simulink model "ATRIAS_vnmc"  (R2015a)
settings: Solver=ode45  StartTime=0.0  StopTime=60  FixedStep=1e-3  MinStep=1e-6  RelTol=1e-3  AbsTol=1e-4
values from neighbouring files (symbols this model uses):
  initial_boom_yaw = initial_boom_yaw + delta_yaw0    [run_model.m]
  max_floor_diff = cost_fun_opts.max_floor_diff    [opt_cmaes.m]    (also in run_model.m; set_all_params_simple.m = 0)
  noise_on_off = cost_fun_opts.noise_on_off    [opt_cmaes.m]    (also in run_model.m; set_all_params_simple.m = 0)
  noise_seed = cost_fun_opts.noise_seed    [opt_cmaes.m]    (also in run_model.m; set_all_params_simple.m = 1)
  noise_variance = cost_fun_opts.noise_variance    [opt_cmaes.m]    (also in run_model.m; set_all_params_simple.m = 0.000174532925199)
  SEA_swing_ctrl_on_off = cost_fun_opts.SEA_swing_ctrl_on_off    [opt_cmaes.m]    (also in run_model.m; set_all_params_simple.m = 0)
  sim_t = simout.twalk    [run_model.m]
  steady_dist = cost_fun_opts.steady_dist    [opt_cmaes.m]    (also in run_model.m; set_all_params_simple.m = 10)
  ts_anim = 0.0333    [run_model.m]
undefined symbols (not defined in the file or in its folder): A1_notch_f1, A2_notch_f1, A_lpf_dtau, A_lpf_velocity, B1_lpf_dtau, B1_lpf_velocity, B1_notch_f1, B2_lpf_dtau, B2_lpf_velocity, B2_notch_f1, b_hmotor, b_leg_spring, b_rotor, base_color_d, boom_color_d, boom_mount_to_center_diagonal, breakaway_friction, c, c_jointstop, com_height_offset, contactThr, coulomb_friction, CtrlPar_theta0, D12_S, D12_T, d_com, ddx_max, ddy_max, delta_phi_max, delta_phi_max_buffer, delta_phi_max_dropoff, delta_phi_min, des_forward_velocity, DS_width, dtau_des_max, dtheta0_vmc, dx0_vmc, dy_max, eref, fblink_color_d, fcut_acceleration, floor_color_d, floor_tile_width, floor_zero_height, FmaxBFSH, FmaxGLU, FmaxHAM, FmaxHFL, FmaxRF, FmaxVAS, FPCtrlPar, friction_linear_zone, g, gain_nodes_sea_torque, gamma_stance_thr, gamma_swing_thr, hip_height, HIP_MTR_MAX_CONT_TORQUE, HIP_MTR_MAX_TORQUE, hshaft_color_d ... (+236)
libraries: sm_lib x280, nesl_utility x174, simulink x114, simulink_extras x58, fl_lib x16, mblibv1 x2, dspswit3 x2
(part 10 of 23)

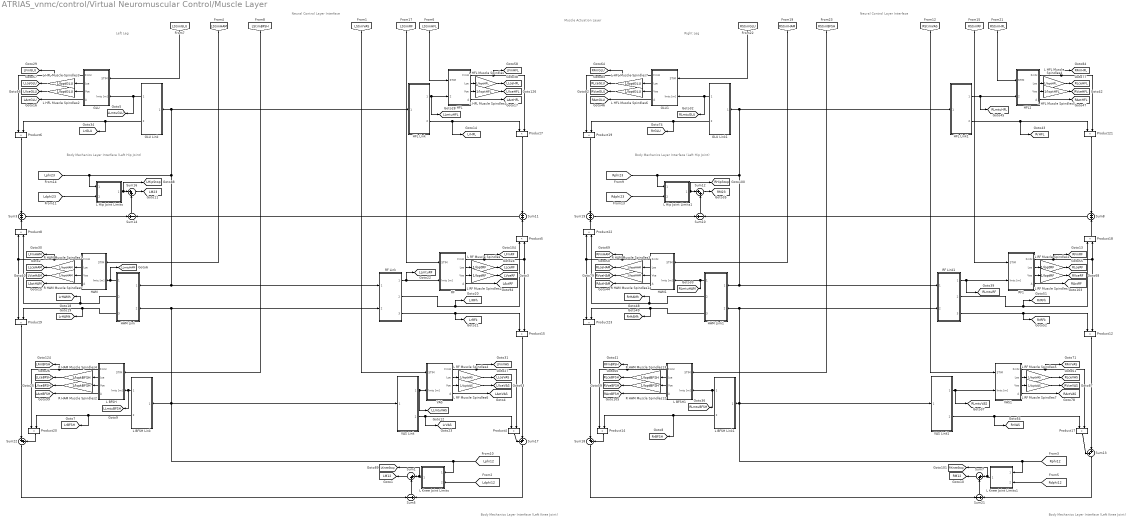
== system ATRIAS_vnmc/control/Virtual Neuromuscular Control/Muscle Layer ==
  note: Left Leg
  note: Neural Control Layer Interface
  note: Muscle Actuation Layer
  note: Body Mechanics Layer
      | Interface (Left Hip Joint)
  note: Body Mechanics Layer
      | Interface (Left Knee Joint)
  note: Right Leg
  note: Neural Control Layer Interface
  note: Body Mechanics Layer
      | Interface (Left Hip Joint)
  note: Body Mechanics Layer
      | Interface (Left Knee Joint)
  GLU : Subsystem
  GLU Link : Subsystem
  GLU Link1 : Subsystem
  GLU1 : Subsystem
  HAM : Subsystem
  HAM Link : Subsystem
  HAM Link1 : Subsystem
  HAM1 : Subsystem
  HFL : Subsystem
  HFL Link : Subsystem
  HFL Link1 : Subsystem
  HFL1 : Subsystem
  L BFSH : Subsystem
  L BFSH Link : Subsystem
  L BFSH Link1 : Subsystem
  L BFSH1 : Subsystem
  L HFL Muscle Spindles{,1,4..5} (4 alike) : Gain  Gain=1/loptHFL
  L HFL Muscle Spindles{2..3,6..7} (4 alike) : Gain  Gain=1/loptGLU
  L Hip Joint Limits : Subsystem
  L Hip Joint Limits1 : Subsystem
  L Knee Joint Limits : Subsystem
  L Knee Joint Limits1 : Subsystem
  L RF Muscle Spindles{,1..3} (4 alike) : Gain  Gain=1/loptRF
  L RF Muscle Spindles{4..7} (4 alike) : Gain  Gain=1/loptVAS
  Product{4..9,12,14..15,17..23} (16 alike) : Product  RndMeth=Zero
  R HAM Muscle Spindles{1,3,6,14} (4 alike) : Gain  Gain=1/loptHAM
  R HAM Muscle Spindles{2,4,12..13} (4 alike) : Gain  Gain=1/loptBFSH
  RF : Subsystem
  RF Link : Subsystem
  RF Link1 : Subsystem
  RF1 : Subsystem
  Sum{1,7,12,16,18,22} (6 alike) : Sum  Inputs=|++
  Sum10 : Sum  Inputs=+-
  Sum{3,8,11,19} (4 alike) : Sum
  Sum13 : Sum  Inputs=++|
  Sum14 : Sum  Inputs=+-
  Sum17 : Sum  Inputs=++|
  Sum21 : Sum  Inputs=-+
  Sum5 : Sum  Inputs=-+
  VAS : Subsystem
  VAS Link : Subsystem
  VAS Link1 : Subsystem
  VAS1 : Subsystem
  tag scope: LActBFSH=global, LActGLU=global, LActHAM=global, LActHFL=global, LActRF=global, LActVAS=global, LFmBFSH=global, LFmGLU=global, LFmHAM=global, LFmHFL=global, LFmRF=global, LFmVAS=global, LHipStop=global, LKneeStop=global, LLceBFSH=global, LLceGLU=global, LLceHAM=global, LLceHFL=global, LLceRF=global, LLceVAS=global, LLmtuBFSH=global, LLmtuGLU=global, LLmtuHAM=global, LLmtuHFL=global, LLmtuRF=global, LLmtuVAS=global, LM12=global, LM23=global, LVceBFSH=global, LVceGLU=global, LVceHAM=global, LVceHFL=global, LVceRF=global, LVceVAS=global, LrBFSH=global, LrGLU=global, LrHAMh=global, LrHAMk=global, LrHFL=global, LrRFh=global, LrRFk=global, LrVAS=global, RActBFSH=global, RActGLU=global, RActHAM=global, RActHFL=global, RActRF=global, RActVAS=global, RFmBFSH=global, RFmGLU=global, RFmHAM=global, RFmHFL=global, RFmRF=global, RFmVAS=global, RHipStop=global, RKneeStop=global, RLceBFSH=global, RLceGLU=global, RLceHAM=global, RLceHFL=global, RLceRF=global, RLceVAS=global, RLmtuBFSH=global, RLmtuGLU=global, RLmtuHAM=global, RLmtuHFL=global, RLmtuRF=global, RLmtuVAS=global, RM12=global, RM23=global, RVceBFSH=global, RVceGLU=global, RVceHAM=global, RVceHFL=global, RVceRF=global, RVceVAS=global, RrBFSH=global, RrGLU=global, RrHAMh=global, RrHAMk=global, RrHFL=global, RrRFh=global, RrRFk=global, RrVAS=global
  wires:
  [Lphi12] -> L Knee Joint Limits/1(phi [rad]1), VAS Link/1(phi23 [rad]), RF Link/2(phi23 [rad]), HAM Link/2(phi23 [rad]), L BFSH Link/1(phi23 [rad])
  [LStimHAM] -> HAM/1(STIM)
  HAM/1(Fmtc) -> Product9/1, Product8/1, [LFmHAM]
  HAM/2(Lce) -> R HAM Muscle Spindles1/1
  HFL/1(Fmtc) -> Product7/2, [LFmHFL]
  HFL/2(Lce) -> L HFL Muscle Spindles/1
  [LStimHFL] -> HFL/1(STIM)
  GLU/1(Fmtc) -> Product6/1, [LFmGLU]
  [LStimGLU] -> GLU/1(STIM)
  Sum16/1 -> [LM23]
  [Ldphi12] -> L Knee Joint Limits/2(dphi [rad/s]1)
  VAS Link/1(lmtu [m]) -> [LLmtuVAS], VAS/2(lmtc [m])
  HAM Link/1(lmtu [m]) -> [LLmtuHAM], HAM/2(lmtc [m])
  HAM Link/2(lever34 [m]) -> Product8/2, [LrHAMh]
  HAM Link/3(lever23 [m]) -> Product9/2, [LrHAMk]
  Sum3/1 -> Sum14/1
  [Lphi23] -> L Hip Joint Limits/1(phi [rad]1), HFL Link/1(phi34 [rad]), GLU Link/1(phi34 [rad]), RF Link/1(phi34 [rad]), HAM Link/1(phi34 [rad])
  VAS/4(A) -> [LActVAS]
  VAS/1(Fmtc) -> Product4/2, [LFmVAS]
  Sum1/1 -> [LM12]
  L Knee Joint Limits/1(M_stop [Nm]1) -> Sum1/1, [LKneeStop]
  Sum5/1 -> Sum1/2
  VAS Link/2(lever [m]) -> [LrVAS], Product4/1
  Sum22/1 -> Sum5/1
  HAM/4(A) -> [LActHAM]
  Product8/1 -> Sum3/2
  Product6/1 -> Sum3/1
  GLU Link/1(lmtu [m]) -> [LLmtuGLU], GLU/2(lmtc [m])
  GLU Link/2(lever [m]) -> Product6/2, [LrGLU]
  GLU/4(A) -> [LActGLU]
  [Ldphi23] -> L Hip Joint Limits/2(dphi [rad/s]1)
  L Hip Joint Limits/1(M_stop [Nm]1) -> [LHipStop], Sum16/1
  Sum14/1 -> Sum16/2
  HFL Link/1(lmtu [m]) -> [LLmtuHFL], HFL/2(lmtc [m])
  HFL/4(A) -> [LActHFL]
  HFL Link/2(lever [m]) -> Product7/1, [LrHFL]
  [LStimVAS] -> VAS/1(STIM)
  GLU/2(Lce) -> L HFL Muscle Spindles3/1
  GLU/3(Vce) -> L HFL Muscle Spindles2/1
  HAM/3(Vce) -> R HAM Muscle Spindles6/1
  VAS/3(Vce) -> L RF Muscle Spindles6/1
  VAS/2(Lce) -> L RF Muscle Spindles4/1
  HFL/3(Vce) -> L HFL Muscle Spindles1/1
  RF/4(A) -> [LActRF]
  RF/3(Vce) -> L RF Muscle Spindles2/1
  RF/2(Lce) -> L RF Muscle Spindles/1
  RF Link/1(lmtu [m]) -> [LLmtuRF], RF/2(lmtc [m])
  RF Link/2(lever34 [m]) -> Product5/1, [LrRFh]
  RF Link/3(lever23 [m]) -> Product15/1, [LrRFk]
  [LStimRF] -> RF/1(STIM)
  Product7/1 -> Sum11/1
  Product5/1 -> Sum11/2
  Product15/1 -> Sum17/2
  Sum17/1 -> Sum5/2
  Product4/1 -> Sum17/1
  [LStimBFSH] -> L BFSH/1(STIM)
  L BFSH Link/1(lmtu [m]) -> [LLmtuBFSH], L BFSH/2(lmtc [m])
  L BFSH Link/2(lever [m]) -> [LrBFSH], Product20/2
  L BFSH/4(A) -> [LActBFSH]
  L BFSH/2(Lce) -> R HAM Muscle Spindles4/1
  L BFSH/3(Vce) -> R HAM Muscle Spindles2/1
  Product20/1 -> Sum22/2
  Product9/1 -> Sum22/1
  L HFL Muscle Spindles1/1 -> [LVceHFL]
  L HFL Muscle Spindles2/1 -> [LVceGLU]
  L HFL Muscle Spindles3/1 -> [LLceGLU]
  L RF Muscle Spindles6/1 -> [LVceVAS]
  RF/1(Fmtc) -> Product5/2, Product15/2, [LFmRF]
  L BFSH/1(Fmtc) -> Product20/1, [LFmBFSH]
  L HFL Muscle Spindles/1 -> [LLceHFL]
  R HAM Muscle Spindles1/1 -> [LLceHAM]
  R HAM Muscle Spindles6/1 -> [LVceHAM]
  L RF Muscle Spindles/1 -> [LLceRF]
  L RF Muscle Spindles2/1 -> [LVceRF]
  R HAM Muscle Spindles4/1 -> [LLceBFSH]
  R HAM Muscle Spindles2/1 -> [LVceBFSH]
  L RF Muscle Spindles4/1 -> [LLceVAS]
  [Rphi12] -> L Knee Joint Limits1/1(phi [rad]1), VAS Link1/1(phi23 [rad]), HAM Link1/2(phi23 [rad]), RF Link1/2(phi23 [rad]), L BFSH Link1/1(phi23 [rad])
  [RStimHAM] -> HAM1/1(STIM)
  HAM1/1(Fmtc) -> Product23/1, Product22/1, [RFmHAM]
  HAM1/2(Lce) -> R HAM Muscle Spindles3/1
  HFL1/1(Fmtc) -> Product21/2, [RFmHFL]
  HFL1/2(Lce) -> L HFL Muscle Spindles4/1
  [RStimHFL] -> HFL1/1(STIM)
  GLU1/1(Fmtc) -> Product19/1, [RFmGLU]
  [RStimGLU] -> GLU1/1(STIM)
  Sum12/1 -> [RM23]
  [Rdphi12] -> L Knee Joint Limits1/2(dphi [rad/s]1)
  VAS Link1/1(lmtu [m]) -> [RLmtuVAS], VAS1/2(lmtc [m])
  HAM Link1/1(lmtu [m]) -> [RLmtuHAM], HAM1/2(lmtc [m])
  HAM Link1/2(lever34 [m]) -> Product22/2, [RrHAMh]
  HAM Link1/3(lever23 [m]) -> Product23/2, [RrHAMk]
  Sum19/1 -> Sum10/1
  [Rphi23] -> L Hip Joint Limits1/1(phi [rad]1), HFL Link1/1(phi34 [rad]), GLU Link1/1(phi34 [rad]), RF Link1/1(phi34 [rad]), HAM Link1/1(phi34 [rad])
  VAS1/4(A) -> [RActVAS]
  VAS1/1(Fmtc) -> Product17/2, [RFmVAS]
  Sum7/1 -> [RM12]
  L Knee Joint Limits1/1(M_stop [Nm]1) -> Sum7/1, [RKneeStop]
  Sum21/1 -> Sum7/2
  VAS Link1/2(lever [m]) -> [RrVAS], Product17/1
  Sum18/1 -> Sum21/1
  HAM1/4(A) -> [RActHAM]
  Product22/1 -> Sum19/2
  Product19/1 -> Sum19/1
  GLU Link1/1(lmtu [m]) -> [RLmtuGLU], GLU1/2(lmtc [m])
  GLU Link1/2(lever [m]) -> Product19/2, [RrGLU]
  GLU1/4(A) -> [RActGLU]
  [Rdphi23] -> L Hip Joint Limits1/2(dphi [rad/s]1)
  L Hip Joint Limits1/1(M_stop [Nm]1) -> [RHipStop], Sum12/1
  Sum10/1 -> Sum12/2
  HFL Link1/1(lmtu [m]) -> [RLmtuHFL], HFL1/2(lmtc [m])
  HFL1/4(A) -> [RActHFL]
  HFL Link1/2(lever [m]) -> Product21/1, [RrHFL]
  [RStimVAS] -> VAS1/1(STIM)
  GLU1/2(Lce) -> L HFL Muscle Spindles7/1
  GLU1/3(Vce) -> L HFL Muscle Spindles6/1
  HAM1/3(Vce) -> R HAM Muscle Spindles14/1
  VAS1/3(Vce) -> L RF Muscle Spindles7/1
  VAS1/2(Lce) -> L RF Muscle Spindles5/1
  HFL1/3(Vce) -> L HFL Muscle Spindles5/1
  RF1/4(A) -> [RActRF]
  RF1/3(Vce) -> L RF Muscle Spindles3/1
  RF1/2(Lce) -> L RF Muscle Spindles1/1
  RF Link1/1(lmtu [m]) -> [RLmtuRF], RF1/2(lmtc [m])
  RF Link1/2(lever34 [m]) -> Product18/1, [RrRFh]
  RF Link1/3(lever23 [m]) -> [RrRFk], Product12/1
  [RStimRF] -> RF1/1(STIM)
  Sum8/1 -> Sum10/2
  Product21/1 -> Sum8/1
  Product18/1 -> Sum8/2
  Product12/1 -> Sum13/2
  Sum13/1 -> Sum21/2
  Product17/1 -> Sum13/1
  [RStimBFSH] -> L BFSH1/1(STIM)
  L BFSH Link1/1(lmtu [m]) -> [RLmtuBFSH], L BFSH1/2(lmtc [m])
  L BFSH Link1/2(lever [m]) -> [RrBFSH], Product14/2
  L BFSH1/4(A) -> [RActBFSH]
  L BFSH1/2(Lce) -> R HAM Muscle Spindles13/1
  L BFSH1/3(Vce) -> R HAM Muscle Spindles12/1
  Product14/1 -> Sum18/2
  Product23/1 -> Sum18/1
  L HFL Muscle Spindles5/1 -> [RVceHFL]
  L HFL Muscle Spindles6/1 -> [RVceGLU]
  L HFL Muscle Spindles7/1 -> [RLceGLU]
  L RF Muscle Spindles7/1 -> [RVceVAS]
  RF1/1(Fmtc) -> Product18/2, Product12/2, [RFmRF]
  L BFSH1/1(Fmtc) -> Product14/1, [RFmBFSH]
  L HFL Muscle Spindles4/1 -> [RLceHFL]
  R HAM Muscle Spindles3/1 -> [RLceHAM]
  R HAM Muscle Spindles14/1 -> [RVceHAM]
  L RF Muscle Spindles1/1 -> [RLceRF]
  L RF Muscle Spindles3/1 -> [RVceRF]
  R HAM Muscle Spindles13/1 -> [RLceBFSH]
  R HAM Muscle Spindles12/1 -> [RVceBFSH]
  L RF Muscle Spindles5/1 -> [RLceVAS]
  Sum11/1 -> Sum14/2

== system ATRIAS_vnmc/control/Virtual Neuromuscular Control/Neural Control Layer1 ==
  note: Neural Control Layer
      | (Sagittal Plane)
  Add{1..3,9} (4 alike) : Sum  Inputs=2
  Add4 : Sum  Inputs=4
  Add5 : Sum  Inputs=4
  Data Type Conversion : DataTypeConversion  OutDataTypeStr=boolean
  Data Type Conversion1 : DataTypeConversion  OutDataTypeStr=boolean
  Demux3 : Demux  Outputs=6
  Demux4 : Demux  Outputs=6
  L Stance Phase (sagittal) : Subsystem  TreatAsAtomicUnit=on
  "L Stance, Swing, Trans (sagittal)" : Subsystem
  L Swing Phase (sagittal) : Subsystem  TreatAsAtomicUnit=on
  Logical Operator : Logic  Operator=NOT  AllPortsSameDT=off  OutDataTypeStr=boolean
  Logical Operator1 : Logic  Operator=NOT  AllPortsSameDT=off  OutDataTypeStr=boolean
  Logical Operator2 : Logic  Operator=OR  AllPortsSameDT=off  OutDataTypeStr=boolean
  Logical Operator3 : Logic  Operator=OR  AllPortsSameDT=off  OutDataTypeStr=boolean
  MDelay{1..4} (4 alike) : Delay  DelayLength=MidDelay_discrete  InitialCondition=0  SampleTime=sample_time
  Mux : Mux  Inputs=6
  Mux1 : Mux  Inputs=6
  Mux2 : Mux  Inputs=2
  Mux4 : Mux  Inputs=2
  R Stance Phase (sagittal) : Subsystem  TreatAsAtomicUnit=on
  "R Stance, Swing, Trans (sagittal)" : Subsystem
  R Swing Phase (sagittal) : Subsystem  TreatAsAtomicUnit=on
  Saturation1 : Saturate  UpperLimit=1  LowerLimit=0.01  ZeroCross=off
  Saturation10 : Saturate  UpperLimit=1  LowerLimit=0.01  ZeroCross=off
  Sum1 : Sum  Inputs=-+|
  Sum6 : Sum  Inputs=-+|
  hipM{1,4,8..9,11..12} (6 alike) : Selector  InputPortWidth=2
  hipM10 : Selector  InputPortWidth=3  Indices=2
  hipM13 : Selector  InputPortWidth=3  Indices=3
  hipM{3,6,14..15,17..18} (6 alike) : Selector  InputPortWidth=2  Indices=2
  hipM16 : Selector  InputPortWidth=3  Indices=3
  hipM2 : Selector  InputPortWidth=3
  hipM5 : Selector  InputPortWidth=3
  hipM7 : Selector  InputPortWidth=3  Indices=2
  tag scope: LAct=global, LHSwStim=global, LStance=global, LStimBFSH=global, LStimGLU=global, LStimHAM=global, LStimHFL=global, LStimRF=global, LStimVAS=global, LSwingPhase=global, RAct=global, RHSwStim=global, RStance=global, RStimBFSH=global, RStimGLU=global, RStimHAM=global, RStimHFL=global, RStimRF=global, RStimVAS=global, RSwingPhase=global
  wires:
  MDelay4/1 -> R Stance Phase (sagittal)/5(FmVAS)
  MDelay3/1 -> L Stance Phase (sagittal)/5(FmVAS)
  [RStance] -> "L Stance, Swing, Trans (sagittal)"/3(CStance)
  [RFootCnt] -> Data Type Conversion1/1
  [LFootCnt] -> Data Type Conversion/1
  [Rphi12] -> R Swing Phase (sagittal)/7(phiK)
  [Rphi23] -> R Swing Phase (sagittal)/6(phiH)
  [Rdphi12] -> R Swing Phase (sagittal)/8(dphiK)
  [Rdalpha] -> R Swing Phase (sagittal)/5(da)
  [Ralpha] -> R Swing Phase (sagittal)/4(a)
  [RLength] -> R Swing Phase (sagittal)/10(l)
  Sum1/1 -> R Swing Phase (sagittal)/3(a_tgt)
  [theta] -> Sum1/1
  [Ralpha_tgt] -> Sum1/2
  [leg_clr] -> R Swing Phase (sagittal)/9(l_clr)
  [Lphi12] -> L Swing Phase (sagittal)/7(phiK)
  [Lphi23] -> L Swing Phase (sagittal)/6(phiH)
  [Ldphi12] -> L Swing Phase (sagittal)/8(dphiK)
  [Ldalpha] -> L Swing Phase (sagittal)/5(da)
  [Lalpha] -> L Swing Phase (sagittal)/4(a)
  [LLength] -> L Swing Phase (sagittal)/10(l)
  Add5/1 -> Mux1/6  "BFSH"
  hipM18/1 -> Add5/4
  hipM17/1 -> Add5/3
  R Swing Phase (sagittal)/3(S_M7_DS [BFSH]) -> Add5/1, "R Stance, Swing, Trans (sagittal)"/14(S_M7_DS)
  hipM16/1 -> Mux1/5  "VAS"
  R Swing Phase (sagittal)/7(M10 [HFL GLU VAS]) -> hipM10/1, hipM2/1, "R Stance, Swing, Trans (sagittal)"/18(S_M10), hipM16/1
  R Swing Phase (sagittal)/5(M8 [RF BFSH]) -> hipM17/1, hipM12/1, "R Stance, Swing, Trans (sagittal)"/16(S_M8)
  R Swing Phase (sagittal)/4(S_M7_Sw [BFSH]) -> Add5/2, "R Stance, Swing, Trans (sagittal)"/15(S_M7_Sw)
  hipM15/1 -> Add4/4
  hipM14/1 -> Add4/3
  L Swing Phase (sagittal)/3(S_M7_DS [BFSH]) -> "L Stance, Swing, Trans (sagittal)"/14(S_M7_DS), Add4/1
  Add4/1 -> Mux/6  "BFSH"
  hipM13/1 -> Mux/5  "VAS"
  "L Stance, Swing, Trans (sagittal)"/2(S_Modules) -> [LAct]
  "R Stance, Swing, Trans (sagittal)"/2(S_Modules) -> [RAct]
  R Swing Phase (sagittal)/8(Phase [M7 M8 M9 M10]) -> [RSwingPhase]
  L Swing Phase (sagittal)/8(Phase [M7 M8 M9 M10]) -> [LSwingPhase]
  hipM11/1 -> Mux1/4  "HAM"
  hipM12/1 -> Mux1/3  "RF"
  Add2/1 -> Mux1/2  "GLU"
  hipM10/1 -> Add2/2
  hipM3/1 -> Add2/1
  Add3/1 -> Mux1/1  "HFL"
  hipM2/1 -> Add3/2
  hipM1/1 -> Add3/1
  Mux1/1 -> [RHSwStim]
  R Swing Phase (sagittal)/6(M9 [HAM BFSH]) -> hipM18/1, hipM11/1, "R Stance, Swing, Trans (sagittal)"/17(S_M9)
  R Swing Phase (sagittal)/2(S_M6 [HFL GLU]) -> hipM1/1, hipM3/1, "R Stance, Swing, Trans (sagittal)"/13(S_M6)
  R Swing Phase (sagittal)/1(S_Sw_0) -> "R Stance, Swing, Trans (sagittal)"/12(S_0_Sw)
  "R Stance, Swing, Trans (sagittal)"/1(S) -> Saturation1/1
  hipM8/1 -> Mux/4  "HAM"
  hipM9/1 -> Mux/3  "RF"
  Add1/1 -> Mux/2  "GLU"
  hipM7/1 -> Add1/2
  hipM6/1 -> Add1/1
  Add9/1 -> Mux/1  "HFL"
  hipM5/1 -> Add9/2
  hipM4/1 -> Add9/1
  Mux/1 -> [LHSwStim]
  L Swing Phase (sagittal)/7(M10 [HFL GLU VAS]) -> hipM7/1, hipM5/1, "L Stance, Swing, Trans (sagittal)"/18(S_M10), hipM13/1
  L Swing Phase (sagittal)/6(M9 [HAM BFSH]) -> hipM8/1, "L Stance, Swing, Trans (sagittal)"/17(S_M9), hipM15/1
  L Swing Phase (sagittal)/5(M8 [RF BFSH]) -> hipM14/1, hipM9/1, "L Stance, Swing, Trans (sagittal)"/16(S_M8)
  L Swing Phase (sagittal)/4(S_M7_Sw [BFSH]) -> "L Stance, Swing, Trans (sagittal)"/15(S_M7_Sw), Add4/2
  L Swing Phase (sagittal)/2(S_M6 [HFL GLU]) -> "L Stance, Swing, Trans (sagittal)"/13(S_M6), hipM4/1, hipM6/1
  L Stance Phase (sagittal)/5(S_M4 [HFL GLU HAM]) -> "L Stance, Swing, Trans (sagittal)"/11(S_M4)
  R Stance Phase (sagittal)/5(S_M4 [HFL GLU HAM]) -> "R Stance, Swing, Trans (sagittal)"/11(S_M4)
  Mux4/1 -> R Stance Phase (sagittal)/3(theta dtheta [rad rad/s])
  Mux2/1 -> L Stance Phase (sagittal)/3(theta dtheta [rad rad/s])
  [RLLoad] -> "R Stance, Swing, Trans (sagittal)"/5(ILLoad)
  R Stance Phase (sagittal)/4(S_M3 [HFL GLU HAM]) -> "R Stance, Swing, Trans (sagittal)"/10(S_M3)
  L Stance Phase (sagittal)/4(S_M3 [HFL GLU HAM]) -> "L Stance, Swing, Trans (sagittal)"/10(S_M3)
  [theta_tgt] -> R Stance Phase (sagittal)/2(theta_tgt [rad])
  [dtheta] -> Mux4/2
  [theta] -> Mux4/1
  [LLLoad] -> "L Stance, Swing, Trans (sagittal)"/5(ILLoad)
  [theta_tgt] -> L Stance Phase (sagittal)/2(theta_tgt [rad])
  [dtheta] -> Mux2/2
  [theta] -> Mux2/1
  R Stance Phase (sagittal)/3(S_M2 [VAS BFSH]) -> "R Stance, Swing, Trans (sagittal)"/9(S_M2)
  R Stance Phase (sagittal)/2(S_M1 [VAS]) -> "R Stance, Swing, Trans (sagittal)"/8(S_M1)
  L Stance Phase (sagittal)/3(S_M2 [VAS BFSH]) -> "L Stance, Swing, Trans (sagittal)"/9(S_M2)
  L Stance Phase (sagittal)/2(S_M1 [VAS]) -> "L Stance, Swing, Trans (sagittal)"/8(S_M1)
  R Stance Phase (sagittal)/1(S_St_0) -> "R Stance, Swing, Trans (sagittal)"/7(S_0_St)
  L Swing Phase (sagittal)/1(S_Sw_0) -> "L Stance, Swing, Trans (sagittal)"/12(S_0_Sw)
  L Stance Phase (sagittal)/1(S_St_0) -> "L Stance, Swing, Trans (sagittal)"/7(S_0_St)
  Sum6/1 -> L Swing Phase (sagittal)/3(a_tgt)
  [LStance] -> "R Stance, Swing, Trans (sagittal)"/3(CStance)
  [RStance] -> "R Stance, Swing, Trans (sagittal)"/2(Stance)
  [LStance] -> "L Stance, Swing, Trans (sagittal)"/2(Stance)
  [theta] -> Sum6/1
  [Lalpha_tgt] -> Sum6/2
  Demux4/6 -> [RStimBFSH]
  Demux4/5 -> [RStimVAS]
  Demux4/4 -> [RStimRF]
  Demux4/3 -> [RStimHAM]
  Demux4/2 -> [RStimGLU]
  Demux4/1 -> [RStimHFL]
  Demux3/6 -> [LStimBFSH]
  Demux3/5 -> [LStimVAS]
  Demux3/4 -> [LStimRF]
  Demux3/3 -> [LStimHAM]
  Demux3/2 -> [LStimGLU]
  Demux3/1 -> [LStimHFL]
  [RLLoad] -> "L Stance, Swing, Trans (sagittal)"/6(CLLoad)
  [LonR] -> "R Stance, Swing, Trans (sagittal)"/4(ConI)
  Saturation1/1 -> Demux4/1
  [LLLoad] -> "R Stance, Swing, Trans (sagittal)"/6(CLLoad)
  [TrCtrlPar] -> "R Stance, Swing, Trans (sagittal)"/1(CtrlPar)
  [LonR] -> Logical Operator2/1
  Logical Operator2/1 -> R Swing Phase (sagittal)/Enable
  Logical Operator1/1 -> Logical Operator2/2
  Data Type Conversion1/1 -> [RStance], R Stance Phase (sagittal)/Enable, Logical Operator1/1, R Swing Phase (sagittal)/2(Stance)
  [SwCtrlPar] -> R Swing Phase (sagittal)/1(CtrlPar)
  [RLceBFSH] -> R Stance Phase (sagittal)/6(LceBFSH)
  MDelay1/1 -> MDelay4/1
  [RFmVAS] -> MDelay1/1
  [LHSwStim] -> R Stance Phase (sagittal)/4(CStim_HSw)
  [StCtrlPar] -> R Stance Phase (sagittal)/1(CtrlPar)
  [RonL] -> "L Stance, Swing, Trans (sagittal)"/4(ConI)
  "L Stance, Swing, Trans (sagittal)"/1(S) -> Saturation10/1
  Saturation10/1 -> Demux3/1
  [TrCtrlPar] -> "L Stance, Swing, Trans (sagittal)"/1(CtrlPar)
  [leg_clr] -> L Swing Phase (sagittal)/9(l_clr)
  [RonL] -> Logical Operator3/1
  Logical Operator3/1 -> L Swing Phase (sagittal)/Enable
  Logical Operator/1 -> Logical Operator3/2
  Data Type Conversion/1 -> [LStance], L Stance Phase (sagittal)/Enable, Logical Operator/1, L Swing Phase (sagittal)/2(Stance)
  [SwCtrlPar] -> L Swing Phase (sagittal)/1(CtrlPar)
  [LLceBFSH] -> L Stance Phase (sagittal)/6(LceBFSH)
  MDelay2/1 -> MDelay3/1
  [LFmVAS] -> MDelay2/1
  [RHSwStim] -> L Stance Phase (sagittal)/4(CStim_HSw)
  [StCtrlPar] -> L Stance Phase (sagittal)/1(CtrlPar)

== system ATRIAS_vnmc/control/Virtual Neuromuscular Control/Torque Distribution ==
  note: J^(-T) [tauB; tauF] = [tauH, tauK]
  note: Map Torques
  note: J^(-T) [tauB; tauF] = [tauH, tauK]
  R tauK_des [Nm] : Inport
  R tauH_des [Nm] : Inport  Port=2
  R Jacobian Constant (k) : Inport  Port=3
  L tauK_des [Nm] : Inport  Port=4
  L tauH_des [Nm] : Inport  Port=5
  L Jacobian Constant (k) : Inport  Port=6
  Demux : Demux
  Demux1 : Demux  Outputs=2
  Demux2 : Demux  Outputs=2
  Mux : Mux
  Mux1 : Mux  Inputs=2
  Mux2 : Mux  Inputs=2
  Switch1 : Switch  Criteria=u2 > Threshold
  Switch2 : Switch  Criteria=u2 > Threshold
  Torque Limiter (outside) 1 : Saturate  UpperLimit=max_sagittal_loaded_torque  LowerLimit=-max_sagittal_loaded_torque
      settings: AttributesFormatString=Hi: %<UpperLimit>\nLo: %<LowerLimit>
  Torque Limiter (outside) 2 : Saturate  UpperLimit=max_sagittal_loaded_torque  LowerLimit=-max_sagittal_loaded_torque
      settings: AttributesFormatString=Hi: %<UpperLimit>\nLo: %<LowerLimit>
  Torque Limiter (outside) 3 : Saturate  UpperLimit=max_sagittal_unloaded_torque  LowerLimit=-max_sagittal_unloaded_torque
      settings: AttributesFormatString=Hi: %<UpperLimit>\nLo: %<LowerLimit>
  Torque Limiter (outside) 4 : Saturate  UpperLimit=max_sagittal_unloaded_torque  LowerLimit=-max_sagittal_unloaded_torque
      settings: AttributesFormatString=Hi: %<UpperLimit>\nLo: %<LowerLimit>
  map_tau_L : MATLAB Function  TreatAsAtomicUnit=on
  map_tau_R : MATLAB Function  TreatAsAtomicUnit=on
  mech limit avoidance1 : Subsystem  Commented=on
  R tauB [Nm] : Outport
  R tauF [Nm] : Outport  Port=2
  R J_inv_transpose [2x2] : Outport  Port=3
  L tauB [Nm] : Outport  Port=4
  L tauF [Nm] : Outport  Port=5
  L J_inv_transpose [2x2] : Outport  Port=6
  wires:
  R Jacobian Constant (k)/1 -> map_tau_R/3(k)
  map_tau_R/3(Jinv_trans) -> R J_inv_transpose [2x2]/1
  L Jacobian Constant (k)/1 -> map_tau_L/3(k)
  map_tau_L/3(Jinv_trans) -> L J_inv_transpose [2x2]/1
  map_tau_L/1(tauB) -> Mux2/1
  map_tau_L/2(tauF) -> Mux2/2
  Mux/1 -> Demux/1
  Demux/1 -> [RtauH]
  R tauH_des [Nm]/1 -> Mux/1
  R tauK_des [Nm]/1 -> Mux/2
  L tauH_des [Nm]/1 -> Mux/3
  L tauK_des [Nm]/1 -> Mux/4
  Demux/2 -> [RtauK]
  Demux/3 -> [LtauH]
  Demux/4 -> [LtauK]
  [RtauH] -> map_tau_R/1(tauH_des)
  [RtauK] -> map_tau_R/2(tauK_des)
  [LtauH] -> map_tau_L/1(tauH_des)
  [LtauK] -> map_tau_L/2(tauK_des)
  Switch1/1 -> Demux1/1
  [LFootCnt] -> Switch1/2
  Mux2/1 -> Torque Limiter (outside) 1/1, Torque Limiter (outside) 3/1
  Torque Limiter (outside) 3/1 -> Switch1/3
  Torque Limiter (outside) 1/1 -> Switch1/1
  Demux1/2 -> L tauF [Nm]/1
  Demux1/1 -> L tauB [Nm]/1
  map_tau_R/1(tauB) -> Mux1/1
  map_tau_R/2(tauF) -> Mux1/2
  Switch2/1 -> Demux2/1
  [RFootCnt] -> Switch2/2
  Mux1/1 -> Torque Limiter (outside) 2/1, Torque Limiter (outside) 4/1
  Torque Limiter (outside) 4/1 -> Switch2/3
  Torque Limiter (outside) 2/1 -> Switch2/1
  Demux2/2 -> R tauF [Nm]/1
  Demux2/1 -> R tauB [Nm]/1

== system ATRIAS_vnmc/atrias_system/ATRIAS Mechanical System Layer/Boom/Frame Data ==
  Mux : Mux  Inputs=3
  PS-Simulink Converter{,1..3} (4 alike) : nesl_utility/PS-Simulink Converter  PhysicalDomain=network_engine_domain  SubClassName=ps_output  LeftPortType=input  RightPortType=output  PseudoPeriodic=off  Frequencies=[]  Unit=1  AffineConversion=off
  Transform Sensor : sm_lib/Frames and Transforms/Transform Sensor  MeasurementFrame=World  SenseAngle=off  SenseAxis=off  SenseAngle1=off  SenseAngle2=off  SenseAngle3=off  SenseQ=on  SenseR=off  SenseOmegaX=off  SenseOmegaY=off  SenseOmegaZ=off  SenseOmega1=off  SenseOmega2=off  SenseOmega3=off  SenseQDot=off  SenseRDot=off  SenseAlphaX=off  SenseAlphaY=off  SenseAlphaZ=off  SenseAlpha1=off  SenseAlpha2=off  SenseAlpha3=off  SenseQDDot=off  SenseRDDot=off  SenseX=on  SenseY=on  SenseZ=on  SenseRad=off  SenseAzim=off  SenseDist=off  SenseInc=off  SenseXDot=off  SenseYDot=off  SenseZDot=off  SenseRadDot=off  SenseAzimDot=off  SenseDistDot=off  SenseIncDot=off  SenseXDDot=off  SenseYDDot=off  SenseZDDot=off  SenseRadDDot=off  SenseAzimDDot=off  SenseDistDDot=off  SenseIncDDot=off  BlockFunction=simmechanics.library.frames_transforms.transform_sensor
  World Frame : sm_lib/Frames and Transforms/World Frame  BlockFunction=simmechanics.library.frames_transforms.world_frame
  Frame : PMIOPort  Port=1  Side=Left
  tag scope: QBoom=global, xyzBoom=global
  wires:
  PS-Simulink Converter/1 -> [QBoom]
  PS-Simulink Converter1/1 -> Mux/1
  PS-Simulink Converter2/1 -> Mux/2
  PS-Simulink Converter3/1 -> Mux/3
  Mux/1 -> [xyzBoom]
  connections:
  Transform Sensor/RConn1 -- Frame/RConn1
  Transform Sensor/LConn1 -- World Frame/RConn1
  Transform Sensor/RConn4 -- PS-Simulink Converter2/LConn1
  Transform Sensor/RConn5 -- PS-Simulink Converter3/LConn1
  Transform Sensor/RConn3 -- PS-Simulink Converter1/LConn1
  Transform Sensor/RConn2 -- PS-Simulink Converter/LConn1

== system ATRIAS_vnmc/atrias_system/ATRIAS Mechanical System Layer/Boom Base/Frame Data ==
  Mux : Mux  Inputs=3
  PS-Simulink Converter{,1..3} (4 alike) : nesl_utility/PS-Simulink Converter  PhysicalDomain=network_engine_domain  SubClassName=ps_output  LeftPortType=input  RightPortType=output  PseudoPeriodic=off  Frequencies=[]  Unit=1  AffineConversion=off
  Transform Sensor : sm_lib/Frames and Transforms/Transform Sensor  MeasurementFrame=World  SenseAngle=off  SenseAxis=off  SenseAngle1=off  SenseAngle2=off  SenseAngle3=off  SenseQ=on  SenseR=off  SenseOmegaX=off  SenseOmegaY=off  SenseOmegaZ=off  SenseOmega1=off  SenseOmega2=off  SenseOmega3=off  SenseQDot=off  SenseRDot=off  SenseAlphaX=off  SenseAlphaY=off  SenseAlphaZ=off  SenseAlpha1=off  SenseAlpha2=off  SenseAlpha3=off  SenseQDDot=off  SenseRDDot=off  SenseX=on  SenseY=on  SenseZ=on  SenseRad=off  SenseAzim=off  SenseDist=off  SenseInc=off  SenseXDot=off  SenseYDot=off  SenseZDot=off  SenseRadDot=off  SenseAzimDot=off  SenseDistDot=off  SenseIncDot=off  SenseXDDot=off  SenseYDDot=off  SenseZDDot=off  SenseRadDDot=off  SenseAzimDDot=off  SenseDistDDot=off  SenseIncDDot=off  BlockFunction=simmechanics.library.frames_transforms.transform_sensor
  World Frame : sm_lib/Frames and Transforms/World Frame  BlockFunction=simmechanics.library.frames_transforms.world_frame
  Frame : PMIOPort  Port=1  Side=Left
  tag scope: QBoomBase=global, xyzBoomBase=global
  wires:
  PS-Simulink Converter/1 -> [QBoomBase]
  PS-Simulink Converter1/1 -> Mux/1
  PS-Simulink Converter2/1 -> Mux/2
  PS-Simulink Converter3/1 -> Mux/3
  Mux/1 -> [xyzBoomBase]
  connections:
  PS-Simulink Converter3/LConn1 -- Transform Sensor/RConn5
  PS-Simulink Converter2/LConn1 -- Transform Sensor/RConn4
  PS-Simulink Converter1/LConn1 -- Transform Sensor/RConn3
  PS-Simulink Converter/LConn1 -- Transform Sensor/RConn2
  Transform Sensor/RConn1 -- Frame/RConn1
  Transform Sensor/LConn1 -- World Frame/RConn1

== system ATRIAS_vnmc/atrias_system/ATRIAS Mechanical System Layer/L Hip Shaft/Frame Data ==
  Mux : Mux  Inputs=3
  PS-Simulink Converter{,1..3} (4 alike) : nesl_utility/PS-Simulink Converter  PhysicalDomain=network_engine_domain  SubClassName=ps_output  LeftPortType=input  RightPortType=output  PseudoPeriodic=off  Frequencies=[]  Unit=1  AffineConversion=off
  Transform Sensor : sm_lib/Frames and Transforms/Transform Sensor  MeasurementFrame=World  SenseAngle=off  SenseAxis=off  SenseAngle1=off  SenseAngle2=off  SenseAngle3=off  SenseQ=on  SenseR=off  SenseOmegaX=off  SenseOmegaY=off  SenseOmegaZ=off  SenseOmega1=off  SenseOmega2=off  SenseOmega3=off  SenseQDot=off  SenseRDot=off  SenseAlphaX=off  SenseAlphaY=off  SenseAlphaZ=off  SenseAlpha1=off  SenseAlpha2=off  SenseAlpha3=off  SenseQDDot=off  SenseRDDot=off  SenseX=on  SenseY=on  SenseZ=on  SenseRad=off  SenseAzim=off  SenseDist=off  SenseInc=off  SenseXDot=off  SenseYDot=off  SenseZDot=off  SenseRadDot=off  SenseAzimDot=off  SenseDistDot=off  SenseIncDot=off  SenseXDDot=off  SenseYDDot=off  SenseZDDot=off  SenseRadDDot=off  SenseAzimDDot=off  SenseDistDDot=off  SenseIncDDot=off  BlockFunction=simmechanics.library.frames_transforms.transform_sensor
  World Frame : sm_lib/Frames and Transforms/World Frame  BlockFunction=simmechanics.library.frames_transforms.world_frame
  Frame : PMIOPort  Port=1  Side=Left
  tag scope: LQHipShaft=global, LxyzHipShaft=global
  wires:
  PS-Simulink Converter/1 -> [LQHipShaft]
  PS-Simulink Converter1/1 -> Mux/1
  PS-Simulink Converter2/1 -> Mux/2
  PS-Simulink Converter3/1 -> Mux/3
  Mux/1 -> [LxyzHipShaft]
  connections:
  Transform Sensor/RConn1 -- Frame/RConn1
  Transform Sensor/LConn1 -- World Frame/RConn1
  Transform Sensor/RConn2 -- PS-Simulink Converter/LConn1
  Transform Sensor/RConn5 -- PS-Simulink Converter3/LConn1
  Transform Sensor/RConn3 -- PS-Simulink Converter1/LConn1
  Transform Sensor/RConn4 -- PS-Simulink Converter2/LConn1

== system ATRIAS_vnmc/atrias_system/ATRIAS Mechanical System Layer/L Leg/Angle Range Map ==
  "[-pi, pi]" : Inport
  Constant : Constant  Value=2*pi
  Sum3 : Sum  Inputs=|++
  Switch : Switch  ZeroCross=off
  "[0,2*pi]" : Outport
  wires:
  "[-pi, pi]"/1 -> Sum3/1, Switch/1, Switch/2
  Sum3/1 -> Switch/3
  Constant/1 -> Sum3/2
  Switch/1 -> "[0,2*pi]"/1

== system ATRIAS_vnmc/atrias_system/ATRIAS Mechanical System Layer/L Leg/Angle Range Map1 ==
  "[-pi, pi]" : Inport
  Constant : Constant  Value=2*pi
  Sum3 : Sum  Inputs=|++
  Switch : Switch  ZeroCross=off
  "[0,2*pi]" : Outport
  wires:
  Switch/1 -> "[0,2*pi]"/1
  Constant/1 -> Sum3/2
  Sum3/1 -> Switch/3
  "[-pi, pi]"/1 -> Switch/2, Switch/1, Sum3/1

== system ATRIAS_vnmc/atrias_system/ATRIAS Mechanical System Layer/L Leg/Four Bar Link ==
  CS1 to CS2 : sm_lib/Frames and Transforms/Rigid Transform  TranslationMethod=Cartesian  TranslationLengthUnit=m  TranslationStandardAxis=+Z  TranslationStandardOffset=0  TranslationCartesianOffset=[0 -l_seg 0]  TranslationROffset=0  TranslationROffsetUnits=m  TranslationZOffset=0  TranslationZOffsetUnits=m  TranslationThetaOffset=0  TranslationThetaOffsetUnits=deg  RotationMethod=None  RotationAngleUnits=deg  RotationStandardAxis=+Z  RotationAngle=0  RotationArbitraryAxis=[0 0 1]  FollAlignAxisA=+X  BaseAlignAxisA=+Y  FollAlignAxisB=+Y  BaseAlignAxisB=+Z  RotationMatrix=[1 0 0; 0 1 0; 0 0 1]  BlockFunction=simmechanics.library.frames_transforms.rigid_transform
  Frame Data : Subsystem
  Solid : sm_lib/Body Elements/Solid  InertiaType=Custom  Mass=m_fblink  MassUnits=kg  CenterOfMass=com_fblink  CenterOfMassUnits=m  MomentsOfInertia=i_fblink_moments  MomentsOfInertiaUnits=kg*m^2  ProductsOfInertia=i_fblink_products  ProductsOfInertiaUnits=kg*m^2  DensityBased=on  Density=1000  DensityUnits=kg/(m^3)  GraphicType=FromGeometry  MarkerShape=Sphere  MarkerSize=10  MarkerSizeUnits=m  GraphicVisPropType=AdvancedVisualProperties  GraphicDiffuseColor=fblink_color_d  GraphicSpecularColor=[0.5 0.5 0.5 1.0]  GraphicAmbientColor=[fblink_color_d*0.5 1.0]  GraphicEmissiveColor=[0.0 0.0 0.0 1.0]  GraphicShininess=128  GraphicOpacity=1.0  GeometryShape=FromFile  RectangleSize=[1 1]  RectangleSizeUnits=m  BrickDimensions=[0.1 l_seg 0.1]  BrickDimensionUnits=m  CylinderRadius=l_rad  CylinderRadiusUnits=m  CylinderLength=l_seg  CylinderLengthUnits=m  SphereRadius=1  SphereRadiusUnits=m  EllipsoidRadii=[1 1 1]  EllipsoidRadiiUnits=m  ExtrusionCrossSection=[1 1; -1 1; -1 -1; 1 -1]  ExtrusionCrossSectionUnits=m  ExtrusionLength=1  ExtrusionLengthUnits=m  PolygonNumSides=3  PolygonOuterRadius=1  PolygonOuterRadiusUnits=m  ExtGeomFileType=STL  ExtGeomFileName=../0_images/models/four_bar_link.stl  ExtGeomFileUnits=m  RevolutionCrossSection=[1 1; 1 -1; 2 -1; 2 1]  RevolutionCrossSectionUnits=m  RevolutionExtent=Full  RevolutionAngle=180  RevolutionAngleUnits=deg  BlockFunction=simmechanics.library.body_elements.solid
  CS1 : PMIOPort  Port=1  Side=Left
  CS2 : PMIOPort  Port=2  Side=Right
  connections:
  CS2/RConn1 -- CS1 to CS2/RConn1
  Solid/RConn1 -- CS1/RConn1 -- Frame Data/LConn1 -- CS1 to CS2/LConn1

== system ATRIAS_vnmc/atrias_system/ATRIAS Mechanical System Layer/L Leg/Lower Leg ==
  CS1 to CS2 : sm_lib/Frames and Transforms/Rigid Transform  TranslationMethod=Cartesian  TranslationLengthUnit=m  TranslationStandardAxis=+Z  TranslationStandardOffset=0  TranslationCartesianOffset=[0 -lowerleg_12 0]  TranslationROffset=0  TranslationROffsetUnits=m  TranslationZOffset=0  TranslationZOffsetUnits=m  TranslationThetaOffset=0  TranslationThetaOffsetUnits=deg  RotationMethod=None  RotationAngleUnits=deg  RotationStandardAxis=+Z  RotationAngle=0  RotationArbitraryAxis=[0 0 1]  FollAlignAxisA=+X  BaseAlignAxisA=+Y  FollAlignAxisB=+Y  BaseAlignAxisB=+Z  RotationMatrix=[1 0 0; 0 1 0; 0 0 1]  BlockFunction=simmechanics.library.frames_transforms.rigid_transform
  CS1 to CS3 : sm_lib/Frames and Transforms/Rigid Transform  TranslationMethod=Cartesian  TranslationLengthUnit=m  TranslationStandardAxis=+Z  TranslationStandardOffset=0  TranslationCartesianOffset=[0 -l_seg 0]  TranslationROffset=0  TranslationROffsetUnits=m  TranslationZOffset=0  TranslationZOffsetUnits=m  TranslationThetaOffset=0  TranslationThetaOffsetUnits=deg  RotationMethod=None  RotationAngleUnits=deg  RotationStandardAxis=+Z  RotationAngle=0  RotationArbitraryAxis=[0 0 1]  FollAlignAxisA=+X  BaseAlignAxisA=+Y  FollAlignAxisB=+Y  BaseAlignAxisB=+Z  RotationMatrix=[1 0 0; 0 1 0; 0 0 1]  BlockFunction=simmechanics.library.frames_transforms.rigid_transform
  Frame Data : Subsystem
  Solid : sm_lib/Body Elements/Solid  InertiaType=Custom  Mass=m_lowerleg  MassUnits=kg  CenterOfMass=com_lowerleg  CenterOfMassUnits=m  MomentsOfInertia=i_lowerleg_moments  MomentsOfInertiaUnits=kg*m^2  ProductsOfInertia=i_lowerleg_products  ProductsOfInertiaUnits=kg*m^2  DensityBased=on  Density=1000  DensityUnits=kg/(m^3)  GraphicType=FromGeometry  MarkerShape=Sphere  MarkerSize=10  MarkerSizeUnits=m  GraphicVisPropType=AdvancedVisualProperties  GraphicDiffuseColor=lowerleg_color_d  GraphicSpecularColor=[0.5 0.5 0.5 1.0]  GraphicAmbientColor=[lowerleg_color_d*0.5 1.0]  GraphicEmissiveColor=[0.0 0.0 0.0 1.0]  GraphicShininess=128  GraphicOpacity=1.0  GeometryShape=FromFile  RectangleSize=[1 1]  RectangleSizeUnits=m  BrickDimensions=[0.1 l_seg 0.1]  BrickDimensionUnits=m  CylinderRadius=l_rad  CylinderRadiusUnits=m  CylinderLength=l_seg  CylinderLengthUnits=m  SphereRadius=1  SphereRadiusUnits=m  EllipsoidRadii=[1 1 1]  EllipsoidRadiiUnits=m  ExtrusionCrossSection=[1 1; -1 1; -1 -1; 1 -1]  ExtrusionCrossSectionUnits=m  ExtrusionLength=1  ExtrusionLengthUnits=m  PolygonNumSides=3  PolygonOuterRadius=1  PolygonOuterRadiusUnits=m  ExtGeomFileType=STL  ExtGeomFileName=../0_images/models/lower_leg.STL  ExtGeomFileUnits=m  RevolutionCrossSection=[1 1; 1 -1; 2 -1; 2 1]  RevolutionCrossSectionUnits=m  RevolutionExtent=Full  RevolutionAngle=180  RevolutionAngleUnits=deg  BlockFunction=simmechanics.library.body_elements.solid
  CS1 : PMIOPort  Port=1  Side=Left
  CS2 : PMIOPort  Port=2  Side=Right
  CS3 : PMIOPort  Port=3  Side=Right
  connections:
  CS3/RConn1 -- CS1 to CS3/RConn1
  Frame Data/LConn1 -- CS1 to CS3/LConn1 -- CS1 to CS2/LConn1 -- Solid/RConn1 -- CS1/RConn1
  CS2/RConn1 -- CS1 to CS2/RConn1

== system ATRIAS_vnmc/atrias_system/ATRIAS Mechanical System Layer/L Leg/Mechanical Limits ==
  note: Thigh-Shin Flexion Collision
  note: Thigh-Shin Collision
  note: Mechanical Limits Model
  dphi_shin : Inport
  phi_shin : Inport  Port=2
  dphi_thigh : Inport  Port=3
  phi_thigh : Inport  Port=4
  Compare To Constant5 : simulink/Logic and Bit Operations/Compare To Constant  relop=<=  const=phi_max_collision  OutDataTypeStr=boolean  ZeroCross=off
  Compare To Zero{,1..5} (6 alike) : simulink/Logic and Bit Operations/Compare To Zero  relop=<=  OutDataTypeStr=boolean  ZeroCross=off
  Constant : Constant  Value=delta_phi_min
  Constant1 : Constant  Value=phi_shin_max
  Constant2 : Constant  Value=phi_thigh_min
  Constant3 : Constant  Value=delta_phi_max
  Constant4 : Constant  Value=phi_shin_min
  Constant5 : Constant  Value=phi_thigh_max
  Enabled Subsystem : Subsystem  TreatAsAtomicUnit=on
  Gain : Gain  Gain=-1
  Gain1 : Gain  Gain=-1
  Gain2 : Gain  Gain=-1
  Logical Operator : Logic  Operator=OR  Inputs=1  AllPortsSameDT=off  OutDataTypeStr=boolean
  Mux : Mux  Inputs=6
  Shin Max Collision Model : Subsystem
  Shin Min Collision Model : Subsystem
  Stop Simulation6 : Stop
  Sum{1..3,5,7} (5 alike) : Sum  Inputs=-+|
  Sum10 : Sum  Inputs=+-|
  Sum11 : Sum  Inputs=-|+
  Sum4 : Sum  Inputs=+-|
  Sum6 : Sum  Inputs=+|-
  Sum8 : Sum  Inputs=+-|
  Sum9 : Sum  Inputs=-|+
  Thigh Max Collision Model : Subsystem
  Thigh Min Collision Model : Subsystem
  Thigh-Shin Collision Model : Subsystem
  Thigh-Shin Collision Model1 : Subsystem
  tau_shin_col : Outport
  tau_thigh_shin_col : Outport  Port=2
  tau_thigh_col : Outport  Port=3
  wires:
  Compare To Constant5/1 -> Logical Operator/1, Enabled Subsystem/1(Col_Flags)
  Sum4/1 -> Shin Max Collision Model/1(phi [rad]), Compare To Zero1/1, [col_r_shin_max]
  Sum10/1 -> [col_r_thigh_max], Compare To Zero5/1, Thigh Max Collision Model/1(phi [rad])
  Logical Operator/1 -> Enabled Subsystem/Enable, Stop Simulation6/1
  Mux/1 -> Compare To Constant5/1
  [col_r_leg_flexion] -> Mux/6
  [col_r_leg_extension] -> Mux/5
  [col_r_shin_min] -> Mux/4
  [col_r_shin_max] -> Mux/3
  [col_r_thigh_min] -> Mux/2
  [col_r_thigh_max] -> Mux/1
  Thigh Max Collision Model/1(tau_interaction[Nm]) -> Sum11/1
  Gain1/1 -> Thigh Max Collision Model/2(vphi [rad/s])
  Thigh Min Collision Model/1(tau_interaction[Nm]) -> Sum11/2
  Sum11/1 -> tau_thigh_col/1
  Compare To Zero5/1 -> Thigh Max Collision Model/Enable
  Constant5/1 -> Sum10/1
  Sum6/1 -> tau_thigh_shin_col/1
  Shin Min Collision Model/1(tau_interaction[Nm]) -> Sum9/2
  Shin Max Collision Model/1(tau_interaction[Nm]) -> Sum9/1
  Sum9/1 -> tau_shin_col/1
  dphi_shin/1 -> Shin Min Collision Model/2(vphi [rad/s]), Gain/1, Sum2/2
  Sum7/1 -> Shin Min Collision Model/1(phi [rad]), Compare To Zero4/1, [col_r_shin_min]
  Constant4/1 -> Sum7/1
  Compare To Zero4/1 -> Shin Min Collision Model/Enable
  Gain2/1 -> Thigh-Shin Collision Model1/2(vphi [rad/s])
  Thigh-Shin Collision Model1/1(tau_interaction[Nm]) -> Sum6/2
  Thigh-Shin Collision Model/1(tau_interaction[Nm]) -> Sum6/1
  Sum8/1 -> Thigh-Shin Collision Model1/1(delta_phi [rad]), Compare To Zero3/1, [col_r_leg_flexion]
  Constant3/1 -> Sum8/1
  Compare To Zero3/1 -> Thigh-Shin Collision Model1/Enable
  Compare To Zero2/1 -> Thigh Min Collision Model/Enable
  Gain/1 -> Shin Max Collision Model/2(vphi [rad/s])
  Sum5/1 -> Thigh Min Collision Model/1(phi [rad]), Compare To Zero2/1, [col_r_thigh_min]
  Constant2/1 -> Sum5/1
  dphi_thigh/1 -> Sum2/1, Gain1/1, Thigh Min Collision Model/2(vphi [rad/s])
  phi_thigh/1 -> Sum1/1, Sum5/2, Sum10/2
  Constant1/1 -> Sum4/1
  Compare To Zero1/1 -> Shin Max Collision Model/Enable
  Sum3/1 -> Thigh-Shin Collision Model/1(delta_phi [rad]), Compare To Zero/1, [col_r_leg_extension]
  Constant/1 -> Sum3/1
  Sum2/1 -> Thigh-Shin Collision Model/2(vphi [rad/s]), Gain2/1
  phi_shin/1 -> Sum4/2, Sum7/2, Sum1/2
  Sum1/1 -> Sum3/2, Sum8/2
  Compare To Zero/1 -> Thigh-Shin Collision Model/Enable

== system ATRIAS_vnmc/atrias_system/ATRIAS Mechanical System Layer/L Leg/Position Sensor ==
  Mux : Mux  Inputs=3
  PS-Simulink Converter1 : nesl_utility/PS-Simulink Converter  PhysicalDomain=network_engine_domain  SubClassName=ps_output  LeftPortType=input  RightPortType=output  PseudoPeriodic=off  Frequencies=[]  Unit=1  AffineConversion=off
  PS-Simulink Converter2 : nesl_utility/PS-Simulink Converter  PhysicalDomain=network_engine_domain  SubClassName=ps_output  LeftPortType=input  RightPortType=output  PseudoPeriodic=off  Frequencies=[]  Unit=1  AffineConversion=off
  PS-Simulink Converter3 : nesl_utility/PS-Simulink Converter  PhysicalDomain=network_engine_domain  SubClassName=ps_output  LeftPortType=input  RightPortType=output  PseudoPeriodic=off  Frequencies=[]  Unit=1  AffineConversion=off
  Transform Sensor : sm_lib/Frames and Transforms/Transform Sensor  MeasurementFrame=World  SenseAngle=off  SenseAxis=off  SenseAngle1=off  SenseAngle2=off  SenseAngle3=off  SenseQ=off  SenseR=off  SenseOmegaX=off  SenseOmegaY=off  SenseOmegaZ=off  SenseOmega1=off  SenseOmega2=off  SenseOmega3=off  SenseQDot=off  SenseRDot=off  SenseAlphaX=off  SenseAlphaY=off  SenseAlphaZ=off  SenseAlpha1=off  SenseAlpha2=off  SenseAlpha3=off  SenseQDDot=off  SenseRDDot=off  SenseX=on  SenseY=on  SenseZ=on  SenseRad=off  SenseAzim=off  SenseDist=off  SenseInc=off  SenseXDot=off  SenseYDot=off  SenseZDot=off  SenseRadDot=off  SenseAzimDot=off  SenseDistDot=off  SenseIncDot=off  SenseXDDot=off  SenseYDDot=off  SenseZDDot=off  SenseRadDDot=off  SenseAzimDDot=off  SenseDistDDot=off  SenseIncDDot=off  BlockFunction=simmechanics.library.frames_transforms.transform_sensor
  World Frame : sm_lib/Frames and Transforms/World Frame  BlockFunction=simmechanics.library.frames_transforms.world_frame
  Frame : PMIOPort  Port=1  Side=Left
  xyz : Outport
  wires:
  PS-Simulink Converter1/1 -> Mux/1
  PS-Simulink Converter2/1 -> Mux/2
  PS-Simulink Converter3/1 -> Mux/3
  Mux/1 -> xyz/1
  connections:
  PS-Simulink Converter3/LConn1 -- Transform Sensor/RConn4
  PS-Simulink Converter2/LConn1 -- Transform Sensor/RConn3
  PS-Simulink Converter1/LConn1 -- Transform Sensor/RConn2
  Transform Sensor/RConn1 -- Frame/RConn1
  Transform Sensor/LConn1 -- World Frame/RConn1

== system ATRIAS_vnmc/atrias_system/ATRIAS Mechanical System Layer/L Leg/Position Sensor1 ==
  Mux : Mux  Inputs=3
  PS-Simulink Converter1 : nesl_utility/PS-Simulink Converter  PhysicalDomain=network_engine_domain  SubClassName=ps_output  LeftPortType=input  RightPortType=output  PseudoPeriodic=off  Frequencies=[]  Unit=1  AffineConversion=off
  PS-Simulink Converter2 : nesl_utility/PS-Simulink Converter  PhysicalDomain=network_engine_domain  SubClassName=ps_output  LeftPortType=input  RightPortType=output  PseudoPeriodic=off  Frequencies=[]  Unit=1  AffineConversion=off
  PS-Simulink Converter3 : nesl_utility/PS-Simulink Converter  PhysicalDomain=network_engine_domain  SubClassName=ps_output  LeftPortType=input  RightPortType=output  PseudoPeriodic=off  Frequencies=[]  Unit=1  AffineConversion=off
  Transform Sensor : sm_lib/Frames and Transforms/Transform Sensor  MeasurementFrame=World  SenseAngle=off  SenseAxis=off  SenseAngle1=off  SenseAngle2=off  SenseAngle3=off  SenseQ=off  SenseR=off  SenseOmegaX=off  SenseOmegaY=off  SenseOmegaZ=off  SenseOmega1=off  SenseOmega2=off  SenseOmega3=off  SenseQDot=off  SenseRDot=off  SenseAlphaX=off  SenseAlphaY=off  SenseAlphaZ=off  SenseAlpha1=off  SenseAlpha2=off  SenseAlpha3=off  SenseQDDot=off  SenseRDDot=off  SenseX=on  SenseY=on  SenseZ=on  SenseRad=off  SenseAzim=off  SenseDist=off  SenseInc=off  SenseXDot=off  SenseYDot=off  SenseZDot=off  SenseRadDot=off  SenseAzimDot=off  SenseDistDot=off  SenseIncDot=off  SenseXDDot=off  SenseYDDot=off  SenseZDDot=off  SenseRadDDot=off  SenseAzimDDot=off  SenseDistDDot=off  SenseIncDDot=off  BlockFunction=simmechanics.library.frames_transforms.transform_sensor
  World Frame : sm_lib/Frames and Transforms/World Frame  BlockFunction=simmechanics.library.frames_transforms.world_frame
  Frame : PMIOPort  Port=1  Side=Left
  xyz : Outport
  wires:
  PS-Simulink Converter1/1 -> Mux/1
  PS-Simulink Converter2/1 -> Mux/2
  PS-Simulink Converter3/1 -> Mux/3
  Mux/1 -> xyz/1
  connections:
  PS-Simulink Converter3/LConn1 -- Transform Sensor/RConn4
  PS-Simulink Converter2/LConn1 -- Transform Sensor/RConn3
  PS-Simulink Converter1/LConn1 -- Transform Sensor/RConn2
  Transform Sensor/RConn1 -- Frame/RConn1
  Transform Sensor/LConn1 -- World Frame/RConn1

== system ATRIAS_vnmc/atrias_system/ATRIAS Mechanical System Layer/L Leg/Shin ==
  CS1 to CS2 : sm_lib/Frames and Transforms/Rigid Transform  TranslationMethod=Cartesian  TranslationLengthUnit=m  TranslationStandardAxis=+Z  TranslationStandardOffset=0  TranslationCartesianOffset=[0 -shin_12 0]  TranslationROffset=0  TranslationROffsetUnits=m  TranslationZOffset=0  TranslationZOffsetUnits=m  TranslationThetaOffset=0  TranslationThetaOffsetUnits=deg  RotationMethod=None  RotationAngleUnits=deg  RotationStandardAxis=+Z  RotationAngle=0  RotationArbitraryAxis=[0 0 1]  FollAlignAxisA=+X  BaseAlignAxisA=+Y  FollAlignAxisB=+Y  BaseAlignAxisB=+Z  RotationMatrix=[1 0 0; 0 1 0; 0 0 1]  BlockFunction=simmechanics.library.frames_transforms.rigid_transform
  Frame Data : Subsystem
  Solid : sm_lib/Body Elements/Solid  InertiaType=Custom  Mass=m_shin  MassUnits=kg  CenterOfMass=com_shin  CenterOfMassUnits=m  MomentsOfInertia=i_shin_moments  MomentsOfInertiaUnits=kg*m^2  ProductsOfInertia=i_shin_products  ProductsOfInertiaUnits=kg*m^2  DensityBased=on  Density=1000  DensityUnits=kg/(m^3)  GraphicType=FromGeometry  MarkerShape=Sphere  MarkerSize=10  MarkerSizeUnits=m  GraphicVisPropType=AdvancedVisualProperties  GraphicDiffuseColor=shin_color_d  GraphicSpecularColor=[0.5 0.5 0.5 1.0]  GraphicAmbientColor=[shin_color_d*0.5 1.0]  GraphicEmissiveColor=[0.0 0.0 0.0 1.0]  GraphicShininess=128  GraphicOpacity=1.0  GeometryShape=FromFile  RectangleSize=[1 1]  RectangleSizeUnits=m  BrickDimensions=[1 1 1]  BrickDimensionUnits=m  CylinderRadius=l_rad  CylinderRadiusUnits=m  CylinderLength=l_seg  CylinderLengthUnits=m  SphereRadius=1  SphereRadiusUnits=m  EllipsoidRadii=[1 1 1]  EllipsoidRadiiUnits=m  ExtrusionCrossSection=[1 1; -1 1; -1 -1; 1 -1]  ExtrusionCrossSectionUnits=m  ExtrusionLength=1  ExtrusionLengthUnits=m  PolygonNumSides=3  PolygonOuterRadius=1  PolygonOuterRadiusUnits=m  ExtGeomFileType=STL  ExtGeomFileName=../0_images/models/shin.STL  ExtGeomFileUnits=m  RevolutionCrossSection=[1 1; 1 -1; 2 -1; 2 1]  RevolutionCrossSectionUnits=m  RevolutionExtent=Full  RevolutionAngle=180  RevolutionAngleUnits=deg  BlockFunction=simmechanics.library.body_elements.solid
  CS1 : PMIOPort  Port=1  Side=Left
  CS2 : PMIOPort  Port=2  Side=Right
  connections:
  CS1 to CS2/LConn1 -- CS1/RConn1 -- Frame Data/LConn1 -- Solid/RConn1
  CS2/RConn1 -- CS1 to CS2/RConn1

== system ATRIAS_vnmc/atrias_system/ATRIAS Mechanical System Layer/L Leg/Shin SEA ==
  note: Shin SEA Mechanics
  Shin Gear Torque [Nm] : Inport
  Shin Joint [rad rad/s] : Inport  Port=2
  Demux : Demux  Outputs=2
  Gain : Gain  Gain=k_leg_spring
  Gain1 : Gain  Gain=b_leg_spring
  Initial Gear Angle : Constant  Value=shin_initial_l
  Inverse Gear Ratio2 : Gain  Gain=1/N_sag
  Inverse Gear Ratio3 : Gain  Gain=Kt_leg
  Inverse Gear Ratio4 : Gain  Gain=1/Kt_leg
  Motor Efficiency : Gain  Gain=mu_motor
  Motor Controller : Subsystem  Commented=on
  Motor Electromagnetism : Subsystem  Commented=on
  Rotor Damping : Gain  Gain=b_rotor
  Rotor and Gearing : Subsystem
  Sum : Sum  Inputs=++|
  Sum2 : Sum  Inputs=+|-
  Sum3 : Sum  Inputs=|+-
  Sum4 : Sum  Inputs=+|-
  Sum5 : Sum  Inputs=|++
  Terminator : Terminator
  Torque Limiter (outside) 2 : Saturate  UpperLimit=LEG_MTR_MAX_TORQUE  LowerLimit=-LEG_MTR_MAX_TORQUE  ZeroCross=off
      settings: AttributesFormatString=Hi: %<UpperLimit>\nLo: %<LowerLimit>
  Rotor Joint Conn : PMIOPort  Port=1  Side=Left
  Shin Joint Torque [Nm] : Outport
  Shin Gear [rad] : Outport  Port=2
  Shin Gear Velocity [rad/s] : Outport  Port=3
  Shin Gear Acceleration [rad/s^2] : Outport  Port=4
  Rotor Stiction [Nm] : Outport  Port=5
  wires:
  Sum2/1 -> Gain/1
  Sum5/1 -> Rotor and Gearing/2(Spring Torque [Nm]), Shin Joint Torque [Nm]/1
  Sum3/1 -> Motor Efficiency/1
  Rotor Damping/1 -> Sum3/2
  Gain/1 -> Sum5/1  "tau_load"
  Gain1/1 -> Sum5/2
  Sum4/1 -> Gain1/1
  Shin Joint [rad rad/s]/1 -> Demux/1
  Demux/1 -> Sum2/2
  Demux/2 -> Sum4/2
  Inverse Gear Ratio3/1 -> Sum3/1
  Initial Gear Angle/1 -> Sum/1
  Sum/1 -> Shin Gear [rad]/1, Sum2/1
  Rotor and Gearing/1(Gearhead Position [rad]) -> Sum/2
  Rotor and Gearing/2(Gearhead Velocity [rad/s]) -> Rotor Damping/1, Shin Gear Velocity [rad/s]/1, Sum4/1
  Motor Efficiency/1 -> Rotor and Gearing/1(Rotor Torque [Nm])
  Inverse Gear Ratio4/1 -> Inverse Gear Ratio3/1
  Motor Controller/1(Voltage [V]) -> Motor Electromagnetism/1(Voltage [V])
  Motor Electromagnetism/1(Current [A]) -> Motor Controller/2(Measured Current [A])
  Shin Gear Torque [Nm]/1 -> Torque Limiter (outside) 2/1
  Inverse Gear Ratio2/1 -> Inverse Gear Ratio4/1
  Rotor and Gearing/5(Rotor Velocity [rad/s]) -> Terminator/1
  Torque Limiter (outside) 2/1 -> Inverse Gear Ratio2/1
  Rotor and Gearing/3(Gearhead Acceleration [rad/s^2]) -> Shin Gear Acceleration [rad/s^2]/1
  Rotor and Gearing/4(Rotor Stiction [Nm]) -> Rotor Stiction [Nm]/1
  connections:
  Rotor and Gearing/LConn1 -- Rotor Joint Conn/RConn1
